simulink model "s3"  (R2022a)
settings: Solver=VariableStepAuto  StartTime=0.0  StopTime=150  RelTol=1e-6
settings Model: Creator=PC  LastModifiedBy=PC

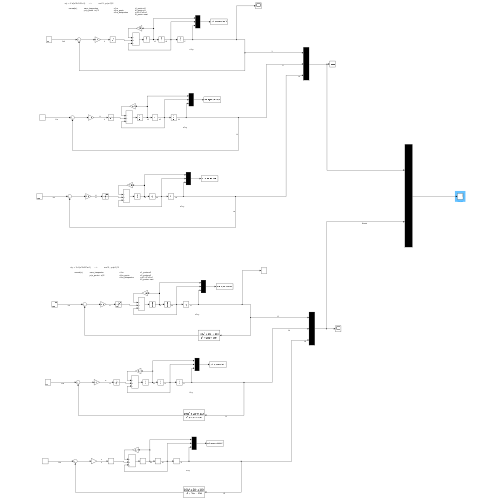
[thumbnail: Simulink's stored preview of the top-level diagram]
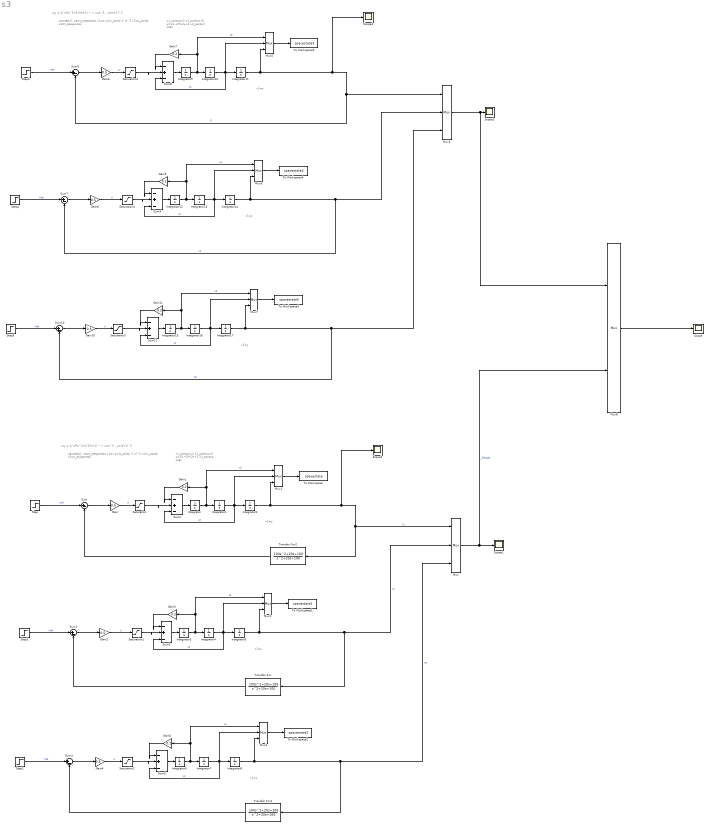
== system s3 ==
  note: x1=y
  note: x1_ponto=x2
      | x2_ponto=x3
      | y=x3 +2*x2+x1
      | x3_ponto= usat
  note: ua=sat(u),             ua=z_trespontos					x1=z
      | 				y=(z_ponto + z)^2					x2=z_ponto
      | 												x3=z_doispontos
  note: u/y = 1/ s*(s^2+0.2*s+1) -- > u=s^3 , y=(s+1)^2
  note: x1=y
  note: x1=y
  note: u/y = 1/ s*(s^2+0.2*s+1) -- > u=s^3 , y=(s+1)^2
  note: ua=sat(u),             ua=z_trespontos					x1=z
      | 				y=(z_ponto + z)^2					x2=z_ponto
      | 												x3=z_doispontos
  note: x1=y
  note: x1=y
  note: x1=y
  note: x1_ponto=x2
      | x2_ponto=x3
      | y=x3 +2*x2+x1
      | x3_ponto= usat
  Gain{,2,4,6,8,10} (6 alike) : Gain  Gain=0.5
  Gain{1,3,5,7,9,11} (6 alike) : Gain  Gain=0.2
  Integrator{,1..17} (18 alike) : Integrator
  Mux{,1..7} (8 alike) : Mux  Inputs=3
  Mux8 : Mux  Inputs=2
  Saturation{,1..5} (6 alike) : Saturate  UpperLimit=0.1  LowerLimit=-0.1
  Scope{,1..4} (5 alike) : Scope
  Step : Step  SampleTime=0
  Step1 : Step  After=4  SampleTime=0
  Step2 : Step  After=8  SampleTime=0
  Step3 : Step  SampleTime=0
  Step4 : Step  After=4  SampleTime=0
  Step5 : Step  After=8  SampleTime=0
  Sum{,1,4,6..7,10} (6 alike) : Sum  Inputs=|+-
  Sum{2..3,5,8..9,11} (6 alike) : Sum  Inputs=|-+-
  To Workspace : ToWorkspace  VariableName=spacestate  SampleTime=-1
  To Workspace1 : ToWorkspace  VariableName=spacestate1  SampleTime=-1
  To Workspace2 : ToWorkspace  VariableName=spacestate2  SampleTime=-1
  To Workspace3 : ToWorkspace  VariableName=spacestate3  SampleTime=-1
  To Workspace4 : ToWorkspace  VariableName=spacestate4  SampleTime=-1
  To Workspace5 : ToWorkspace  VariableName=spacestate5  SampleTime=-1
  Transfer Fcn : TransferFcn  Numerator=[100 20 100]  Denominator=[1 20 100]
  Transfer Fcn1 : TransferFcn  Numerator=[100 20 100]  Denominator=[1 20 100]
  Transfer Fcn2 : TransferFcn  Numerator=[100 20 100]  Denominator=[1 20 100]
  wires:
  Step/1 -> Sum/1  "Yref"
  Sum/1 -> Gain/1
  Gain/1 -> Saturation/1  "U"
  Integrator/1 -> Mux1/1, Gain1/1, Integrator1/1  "x3"
  Integrator1/1 -> Sum2/3, Integrator2/1, Mux1/2  "x2"
  Integrator2/1 -> Mux1/3, Scope2/1, Mux/1, Transfer Fcn2/1  "Y1"
  Mux1/1 -> To Workspace/1
  Sum2/1 -> Integrator/1
  Gain1/1 -> Sum2/1
  Mux/1 -> Mux8/2, Scope1/1  "_filtrado"
  Integrator4/1 -> Sum3/3, Integrator5/1, Mux2/2  "x2"
  Mux2/1 -> To Workspace1/1
  Sum1/1 -> Gain2/1
  Gain2/1 -> Saturation1/1  "U"
  Integrator3/1 -> Mux2/1, Gain3/1, Integrator4/1  "x3"
  Gain3/1 -> Sum3/1
  Integrator5/1 -> Mux2/3, Transfer Fcn/1, Mux/2  "Y4"
  Step1/1 -> Sum1/1  "Yref"
  Sum3/1 -> Integrator3/1
  Integrator7/1 -> Sum5/3, Integrator8/1, Mux3/2  "x2"
  Mux3/1 -> To Workspace2/1
  Sum4/1 -> Gain4/1
  Gain4/1 -> Saturation2/1  "U"
  Integrator6/1 -> Mux3/1, Gain5/1, Integrator7/1  "x3"
  Gain5/1 -> Sum5/1
  Integrator8/1 -> Mux3/3, Mux/3, Transfer Fcn1/1  "Y8"
  Step2/1 -> Sum4/1  "Yref"
  Sum5/1 -> Integrator6/1
  Saturation/1 -> Sum2/2
  Saturation1/1 -> Sum3/2
  Saturation2/1 -> Sum5/2
  Transfer Fcn/1 -> Sum1/2
  Transfer Fcn1/1 -> Sum4/2
  Transfer Fcn2/1 -> Sum/2
  Integrator10/1 -> Sum8/3, Integrator11/1, Mux5/2  "x2"
  Mux5/1 -> To Workspace3/1
  Sum6/1 -> Gain6/1
  Integrator9/1 -> Mux5/1, Gain7/1, Integrator10/1  "x3"
  Gain6/1 -> Saturation3/1  "U"
  Gain10/1 -> Saturation5/1  "U"
  Mux4/1 -> Mux8/1, Scope3/1
  Integrator11/1 -> Mux5/3, Scope4/1, Sum6/2, Mux4/1  "Y1"
  Sum7/1 -> Gain8/1
  Sum8/1 -> Integrator9/1
  Sum11/1 -> Integrator15/1
  Step5/1 -> Sum10/1  "Yref"
  Integrator17/1 -> Mux7/3, Sum10/2, Mux4/3  "Y8"
  Gain11/1 -> Sum11/1
  Mux7/1 -> To Workspace5/1
  Step3/1 -> Sum6/1  "Yref"
  Saturation3/1 -> Sum8/2
  Integrator14/1 -> Mux6/3, Sum7/2, Mux4/2  "Y4"
  Saturation5/1 -> Sum11/2
  Step4/1 -> Sum7/1  "Yref"
  Sum10/1 -> Gain10/1
  Gain7/1 -> Sum8/1
  Sum9/1 -> Integrator12/1
  Integrator16/1 -> Sum11/3, Integrator17/1, Mux7/2  "x2"
  Gain8/1 -> Saturation4/1  "U"
  Gain9/1 -> Sum9/1
  Integrator12/1 -> Mux6/1, Gain9/1, Integrator13/1  "x3"
  Integrator13/1 -> Sum9/3, Integrator14/1, Mux6/2  "x2"
  Integrator15/1 -> Mux7/1, Gain11/1, Integrator16/1  "x3"
  Mux6/1 -> To Workspace4/1
  Saturation4/1 -> Sum9/2
  Mux8/1 -> Scope/1
